simulink model "chibiOS_Config_Model"  (R2012b)
settings: Solver=FixedStepDiscrete  SolverMode=MultiTasking  StartTime=0.0  StopTime=10.0  FixedStep=0.01  RelTol=1e-3
undefined symbols (not defined in the file or in its folder): chSysHalt, STM32_DMA_STREAM_ID
libraries: lib_ChibiOS x5
settings Model: BufferReuse=off  Creator=freyjed  LastModifiedBy=freyjed
settings OptimizationCC: BlockReduction=off  ConditionallyExecuteInputs=off  BufferReuse=off  OptimizeModelRefInitCode=on  LifeSpan=1
settings HardwareCC: ProdLargestAtomicInteger=Integer  ProdLargestAtomicFloat=Float  ProdIntDivRoundTo=Zero  ProdEndianess=LittleEndian  ProdHWDeviceType=STMicroelectronics->STM32F4xx 32-bit Cortex-M4  TargetLargestAtomicInteger=Integer  TargetLargestAtomicFloat=Float  TargetIntDivRoundTo=Zero  TargetEndianess=LittleEndian  TargetHWDeviceType=ChibiOS->ChibiOS
settings ModelReferenceCC: UpdateModelReferenceTargets=Force
settings RTWCC: SystemTargetFile=ChibiOS.tlc  TemplateMakefile=ChibiOS.tmf  Description=ChibiOS/RT (Embedded RTOS Target)  RetainRTWFile=on  ProcessScript=ChibiOS_make_rtw_hook
settings CodeAppCC: ForceParamTrailComments=on  IgnoreCustomStorageClasses=off  OperatorAnnotations=on  SimulinkDataObjDesc=on  SFDataObjDesc=on  MATLABFcnDesc=on  DefineNamingRule=UpperCase  InsertBlockDesc=on  MATLABSourceComments=on  ReqsInCode=on
settings STFCustomTargetCC: CodeReplacementLibrary=ANSI_C  ModelReferenceCompliant=off  IncludeMdlTerminateFcn=off  CombineOutputUpdateFcns=on  ERTCustomFileBanners=on  SupportContinuousTime=off  SupportNonInlinedSFcns=off  ParenthesesLevel=Maximum  GRTInterface=off  SystemTargetFile=ChibiOS.tlc
settings ERTTargetCC: CodeReplacementLibrary=ANSI_C  MultiwordLength=2048  ModelReferenceCompliant=off  ParMdlRefBuildCompliant=off  CompOptLevelCompliant=off  ConcurrentExecutionCompliant=off  IncludeMdlTerminateFcn=off  ERTFirstTimeCompliant=off  ParenthesesLevel=Maximum  ModelStepFunctionPrototypeControlCompliant=off  CPPClassGenCompliant=off  InlinedParameterPlacement=NonHierarchical  ERTSrcFileBannerTemplate=chibiOS_sourceFileTemplate.cgt  ERTHdrFileBannerTemplate=chibiOS_sourceFileTemplate.cgt  ERTDataSrcFileTemplate=chibiOS_sourceFileTemplate.cgt  ERTDataHdrFileTemplate=chibiOS_sourceFileTemplate.cgt  ERTCustomFileTemplate=chibiOS_customRoutineProcess.tlc  PreserveExpressionOrder=on  PreserveIfCondition=on  SuppressUnreachableDefaultCases=off

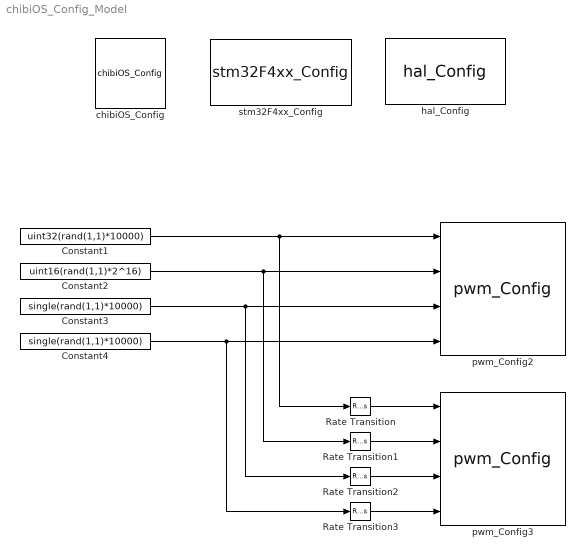
== system chibiOS_Config_Model ==
  Constant1 : Constant  Value=uint32(rand(1,1)*10000)  OutDataTypeStr=uint32
  Constant2 : Constant  Value=uint16(rand(1,1)*2^16)  OutDataTypeStr=uint16
  Constant3 : Constant  Value=single(rand(1,1)*10000)  OutDataTypeStr=single
  Constant4 : Constant  Value=single(rand(1,1)*10000)  OutDataTypeStr=single
  Rate Transition{,1..3} (4 alike) : RateTransition  Integrity=off
  chibiOS_Config : lib_ChibiOS/chibiOS_Config  CH_FREQUENCY=1000  CH_TIME_QUANTUM=20  CH_MEMCORE_SIZE=0  CH_NO_IDLE_THREAD=off  CH_OPTIMIZE_SPEED=on  CH_USE_REGISTRY=on  CH_USE_WAITEXIT=on  CH_USE_SEMAPHORES=on  CH_USE_SEMAPHORES_PRIORITY=off  CH_USE_SEMSW=on  CH_USE_MUTEXES=on  CH_USE_CONDVARS=on  CH_USE_CONDVARS_TIMEOUT=on  CH_USE_EVENTS=on  CH_USE_EVENTS_TIMEOUT=on  CH_USE_MESSAGES=on  CH_USE_MESSAGES_PRIORITY=off  CH_USE_MAILBOXES=on  CH_USE_QUEUES=on  CH_USE_MEMCORE=on  CH_USE_HEAP=on  CH_USE_MALLOC_HEAP=off  CH_USE_MEMPOOLS=on  CH_USE_DYNAMIC=on  CH_DBG_SYSTEM_STATE_CHECK=on  CH_DBG_ENABLE_CHECKS=on  CH_DBG_ENABLE_ASSERTS=on  CH_DBG_ENABLE_TRACE=on  CH_DBG_ENABLE_STACK_CHECK=on  CH_DBG_FILL_THREADS=on  CH_DBG_THREADS_PROFILING=on
  hal_Config : lib_ChibiOS/hal_Config  HAL_USE_TM=on  HAL_USE_PAL=on  HAL_USE_ADC=off  HAL_USE_CAN=off  HAL_USE_EXT=off  HAL_USE_GPT=off  HAL_USE_I2C=off  HAL_USE_ICU=off  HAL_USE_MAC=off  HAL_USE_MMC_SPI=off  HAL_USE_PWM=on  HAL_USE_RTC=off  HAL_USE_SDC=off  HAL_USE_SERIAL=off  HAL_USE_SERIAL_USB=off  HAL_USE_SPI=on  HAL_USE_UART=off  HAL_USE_USB=off  ADC_USE_WAIT=on  ADC_USE_MUTUAL_EXCLUSION=on  CAN_USE_SLEEP_MODE=on  I2C_USE_MUTUAL_EXCLUSION=on  MAC_USE_ZERO_COPY=off  MAC_USE_EVENTS=on  MMC_NICE_WAITING=on  SDC_INIT_RETRY=100  SDC_MMC_SUPPORT=off  SDC_NICE_WAITING=on  SERIAL_DEFAULT_BITRATE=38400  SERIAL_BUFFERS_SIZE=16  SPI_USE_WAIT=on  SPI_USE_MUTUAL_EXCLUSION=off
  pwm_Config2 : lib_ChibiOS/pwm_Config  pwmDriver=3  pwmClockFreq=10000  pwmPeriod=1  pwmChan1=Active High  pwmChan2=Active High  pwmChan3=Active High  pwmChan4=Active High  Ts_pwm=0.5
  pwm_Config3 : lib_ChibiOS/pwm_Config  pwmDriver=4  pwmClockFreq=10000  pwmPeriod=1  pwmChan1=Active High  pwmChan2=Active High  pwmChan3=Active High  pwmChan4=Active High  Ts_pwm=[2 1]
  stm32F4xx_Config : lib_ChibiOS/stm32F4xx_Config  STM32_NO_INIT=off  STM32_HSI_ENABLED=on  STM32_LSI_ENABLED=on  STM32_HSE_ENABLED=on  STM32_LSE_ENABLED=off  STM32_CLOCK48_REQUIRED=on  STM32_SW=Phase locked Loop (PLL)  STM32_PLLSRC=External High Speed Clock (HSE)  STM32_PLLM_VALUE=8  STM32_PLLN_VALUE=336  STM32_PLLP_VALUE=2  STM32_PLLQ_VALUE=7  STM32_HPRE=1  STM32_PPRE1=4  STM32_PPRE2=2  STM32_RTCSEL=LSI  STM32_RTCPRE_VALUE=8  STM32_MCO1SEL=HSI clock on MCO1 pin  STM32_MCO1PRE=1  STM32_MCO2SEL=SYSCLK clock on MCO2 pin  STM32_MCO2PRE=5  STM32_I2SSRC=CKIN  STM32_PLLI2SN_VALUE=192  STM32_PLLI2SR_VALUE=5  STM32_VOS=STM32_VOS_HIGH  STM32_PVD_ENABLE=off  STM32_PLS=Level 0: 214/204 mV  STM32_ADC_ADCPRE=2  STM32_ADC_IRQ_PRIORITY=6  STM32_ADC_USE_ADC1=off  STM32_ADC_ADC1_DMA_STREAM=STM32_DMA_STREAM_ID(2, 4)  STM32_ADC_ADC1_DMA_PRIORITY=2  STM32_ADC_ADC1_DMA_IRQ_PRIORITY=6  STM32_ADC_USE_ADC2=off  STM32_ADC_ADC2_DMA_STREAM=STM32_DMA_STREAM_ID(2, 3)  STM32_ADC_ADC2_DMA_PRIORITY=2  STM32_ADC_ADC2_DMA_IRQ_PRIORITY=6  STM32_ADC_USE_ADC3=off  STM32_ADC_ADC3_DMA_STREAM=STM32_DMA_STREAM_ID(2, 1)  STM32_ADC_ADC3_DMA_PRIORITY=2  STM32_ADC_ADC3_DMA_IRQ_PRIORITY=6  STM32_CAN_USE_CAN1=off  STM32_CAN_CAN1_IRQ_PRIORITY=11  STM32_CAN_USE_CAN2=off  STM32_CAN_CAN2_IRQ_PRIORITY=11  STM32_EXT_EXTI0_IRQ_PRIORITY=10  STM32_EXT_EXTI1_IRQ_PRIORITY=10  STM32_EXT_EXTI2_IRQ_PRIORITY=10  STM32_EXT_EXTI3_IRQ_PRIORITY=10  STM32_EXT_EXTI4_IRQ_PRIORITY=10  STM32_EXT_EXTI5_9_IRQ_PRIORITY=10  STM32_EXT_EXTI10_15_IRQ_PRIORITY=10  STM32_EXT_EXTI16_IRQ_PRIORITY=10  STM32_EXT_EXTI17_IRQ_PRIORITY=1  STM32_EXT_EXTI18_IRQ_PRIORITY=10  STM32_EXT_EXTI19_IRQ_PRIORITY=10  STM32_EXT_EXTI20_IRQ_PRIORITY=10  STM32_EXT_EXTI21_IRQ_PRIORITY=1  STM32_EXT_EXTI22_IRQ_PRIORITY=1  STM32_GPT_USE_TIM1=off  STM32_GPT_TIM1_IRQ_PRIORITY=9  STM32_GPT_USE_TIM2=off  STM32_GPT_TIM2_IRQ_PRIORITY=9  STM32_GPT_USE_TIM3=off  STM32_GPT_TIM3_IRQ_PRIORITY=9  STM32_GPT_USE_TIM4=off  STM32_GPT_TIM4_IRQ_PRIORITY=9  STM32_GPT_USE_TIM5=off  STM32_GPT_TIM5_IRQ_PRIORITY=9  STM32_GPT_USE_TIM6=off  STM32_GPT_TIM6_IRQ_PRIORITY=9  STM32_GPT_USE_TIM7=off  STM32_GPT_TIM7_IRQ_PRIORITY=9  STM32_GPT_USE_TIM8=off  STM32_GPT_TIM8_IRQ_PRIORITY=9  STM32_GPT_USE_TIM9=off  STM32_GPT_TIM9_IRQ_PRIORITY=9  STM32_GPT_USE_TIM11=off  STM32_GPT_TIM11_IRQ_PRIORITY=9  STM32_GPT_USE_TIM12=off  STM32_GPT_TIM12_IRQ_PRIORITY=9  STM32_GPT_USE_TIM14=off  STM32_GPT_TIM14_IRQ_PRIORITY=9  STM32_I2C_USE_I2C1=off  STM32_I2C_I2C1_RX_DMA_STREAM=STM32_DMA_STREAM_ID(1, 0)  STM32_I2C_I2C1_TX_DMA_STREAM=STM32_DMA_STREAM_ID(1, 6)  STM32_I2C_I2C1_IRQ_PRIORITY=11  STM32_I2C_I2C1_DMA_PRIORITY=3  STM32_I2C_I2C1_DMA_ERROR_HOOK=chSysHalt()  STM32_I2C_USE_I2C2=off  STM32_I2C_I2C2_RX_DMA_STREAM=STM32_DMA_STREAM_ID(1, 2)  STM32_I2C_I2C2_TX_DMA_STREAM=STM32_DMA_STREAM_ID(1, 7)  STM32_I2C_I2C2_IRQ_PRIORITY=11  STM32_I2C_I2C2_DMA_PRIORITY=3  STM32_I2C_I2C2_DMA_ERROR_HOOK=chSysHalt()  STM32_I2C_USE_I2C3=off  STM32_I2C_I2C3_RX_DMA_STREAM=STM32_DMA_STREAM_ID(1, 2)  STM32_I2C_I2C3_TX_DMA_STREAM=STM32_DMA_STREAM_ID(1, 4)  STM32_I2C_I2C3_IRQ_PRIORITY=11  STM32_I2C_I2C3_DMA_PRIORITY=3  STM32_I2C_I2C3_DMA_ERROR_HOOK=chSysHalt()  STM32_ICU_USE_TIM1=off  STM32_ICU_TIM1_IRQ_PRIORITY=9  STM32_ICU_USE_TIM2=off  STM32_ICU_TIM2_IRQ_PRIORITY=9  STM32_ICU_USE_TIM3=off  STM32_ICU_TIM3_IRQ_PRIORITY=9  STM32_ICU_USE_TIM4=off  STM32_ICU_TIM4_IRQ_PRIORITY=9  STM32_ICU_USE_TIM5=off  STM32_ICU_TIM5_IRQ_PRIORITY=9  STM32_ICU_USE_TIM8=off  STM32_ICU_TIM8_IRQ_PRIORITY=9  STM32_ICU_USE_TIM9=off  STM32_ICU_TIM9_IRQ_PRIORITY=9  STM32_MAC_TRANSMIT_BUFFERS=2  STM32_MAC_RECEIVE_BUFFERS=4  STM32_MAC_BUFFERS_SIZE=1522  STM32_MAC_PHY_TIMEOUT=100  STM32_MAC_ETH1_CHANGE_PHY_STATE=on  STM32_MAC_ETH1_IRQ_PRIORITY=13  STM32_MAC_IP_CHECKSUM_OFFLOAD=0  STM32_PWM_USE_ADVANCED=off  STM32_PWM_USE_TIM1=off  STM32_PWM_TIM1_IRQ_PRIORITY=9  STM32_PWM_USE_TIM2=off  STM32_PWM_TIM2_IRQ_PRIORITY=9  STM32_PWM_USE_TIM3=on  STM32_PWM_TIM3_IRQ_PRIORITY=9  STM32_PWM_USE_TIM4=on  STM32_PWM_TIM4_IRQ_PRIORITY=9  STM32_PWM_USE_TIM5=off  STM32_PWM_TIM5_IRQ_PRIORITY=9  STM32_PWM_USE_TIM8=off  STM32_PWM_TIM8_IRQ_PRIORITY=9  STM32_PWM_USE_TIM9=off  STM32_PWM_TIM9_IRQ_PRIORITY=9  STM32_SERIAL_USE_USART1=off  STM32_SERIAL_USART1_PRIORITY=4  STM32_SERIAL_USE_USART2=off  STM32_SERIAL_USART2_PRIORITY=4  STM32_SERIAL_USE_USART3=off  STM32_SERIAL_USART3_PRIORITY=4  STM32_SERIAL_USE_UART4=off  STM32_SERIAL_UART4_PRIORITY=4  STM32_SERIAL_USE_UART5=off  STM32_SERIAL_UART5_PRIORITY=4  STM32_SERIAL_USE_USART6=off  STM32_SERIAL_USART6_PRIORITY=4  STM32_SPI_USE_SPI1=off  STM32_SPI_SPI1_RX_DMA_STREAM=STM32_DMA_STREAM_ID(2,0)  STM32_SPI_SPI1_TX_DMA_STREAM=STM32_DMA_STREAM_ID(2,3)  STM32_SPI_SPI1_DMA_PRIORITY=2  STM32_SPI_SPI1_IRQ_PRIORITY=6  STM32_SPI_USE_SPI2=off  STM32_SPI_SPI2_RX_DMA_STREAM=STM32_DMA_STREAM_ID(1,3)  STM32_SPI_SPI2_TX_DMA_STREAM=STM32_DMA_STREAM_ID(1,4)  STM32_SPI_SPI2_DMA_PRIORITY=2  STM32_SPI_SPI2_IRQ_PRIORITY=6  STM32_SPI_USE_SPI3=on  STM32_SPI_SPI3_RX_DMA_STREAM=STM32_DMA_STREAM_ID(1,0)  STM32_SPI_SPI3_TX_DMA_STREAM=STM32_DMA_STREAM_ID(1,7)  STM32_SPI_SPI3_DMA_PRIORITY=2  STM32_SPI_SPI3_IRQ_PRIORITY=6  STM32_SPI_DMA_ERROR_HOOK=chSysHalt()  STM32_UART_USE_USART1=off  STM32_UART_USART1_RX_DMA_STREAM=STM32_DMA_STREAM_ID(2, 5)  STM32_UART_USART1_TX_DMA_STREAM=STM32_DMA_STREAM_ID(2, 7)  STM32_UART_USART1_IRQ_PRIORITY=4  STM32_UART_USART1_DMA_PRIORITY=1  STM32_UART_USE_USART2=off  STM32_UART_USART2_RX_DMA_STREAM=STM32_DMA_STREAM_ID(1, 5)  STM32_UART_USART2_TX_DMA_STREAM=STM32_DMA_STREAM_ID(1, 6)  STM32_UART_USART2_IRQ_PRIORITY=4  STM32_UART_USART2_DMA_PRIORITY=1  STM32_UART_USE_USART3=off  STM32_UART_USART3_RX_DMA_STREAM=STM32_DMA_STREAM_ID(1, 1)  STM32_UART_USART3_TX_DMA_STREAM=STM32_DMA_STREAM_ID(1, 3)  STM32_UART_USART3_IRQ_PRIORITY=4  STM32_UART_USART3_DMA_PRIORITY=1  STM32_UART_USE_USART6=off  STM32_UART_USART6_RX_DMA_STREAM=STM32_DMA_STREAM_ID(2, 2)  STM32_UART_USART6_TX_DMA_STREAM=STM32_DMA_STREAM_ID(2, 7)  STM32_UART_USART6_IRQ_PRIORITY=4  STM32_UART_USART6_DMA_PRIORITY=1  STM32_UART_DMA_ERROR_HOOK=chSysHalt()  STM32_USB_USE_OTG1=off  STM32_USB_OTG1_IRQ_PRIORITY=2  STM32_USB_OTG1_RX_FIFO_SIZE=512  STM32_USB_USE_OTG2=off  STM32_USB_OTG2_IRQ_PRIORITY=2  STM32_USB_OTG2_RX_FIFO_SIZE=1024  STM32_USB_OTG_THREAD_PRIO=LOWPRIO  STM32_USB_OTG_THREAD_STACK_SIZE=128  STM32_USB_OTGFIFO_FILL_BASEPRI=0
  wires:
  Constant1/1 -> pwm_Config2/1, Rate Transition/1
  Constant2/1 -> pwm_Config2/2, Rate Transition1/1
  Constant4/1 -> pwm_Config2/4, Rate Transition3/1
  Constant3/1 -> pwm_Config2/3, Rate Transition2/1
  Rate Transition/1 -> pwm_Config3/1
  Rate Transition1/1 -> pwm_Config3/2
  Rate Transition2/1 -> pwm_Config3/3
  Rate Transition3/1 -> pwm_Config3/4
